simulink library "powerlib2"  (Simulink 6.0)
settings: Solver=ode45  SolverMode=SingleTasking  StartTime=0.0  StopTime=10.0  RelTol=1e-3
undefined symbols (not defined in the file or in its folder): com, ctrl1, Da, DiscIntNeverNeededParam, dtha, etat, FA, gcbh, Ha, Ka, Lm, Ls, powericonV2, q0, Rm, Rs, sel, st_a, st_b, st_c, sta, stb, stc, T1, T2, T3, T4
libraries: powerlib2 x55, simulink_extras x5, powerlib_extras x4, powerlib_modelsV2 x4, simulink x1
(part 3 of 6)

== system powerlib2/Machines ==
  note: ____ S y n c h r o n o u s M a c h i n e s ____________________
  note: ____ D C M a c h i n e s _______________________
  note: ____ A s y n c h r o n o u s M a c h i n e s ___________________
  note: ____ P r i m e M o v e r s a n d R e g u l a t o r s _____
  note: ____ M a c h i n e M e a s u r e m e n t s ___________
  Asynchronous Machine SI Units : Subsystem  Tag=PoWeRsYsTeMbLoCk  LoadFcn=powericonV2('psblfblk',bdroot,'gotofrom','Load');  mask(Asynchronous Machine){rotType=Wound, ctrl=Rotor, x1=[ 3*746, 220, 60 ], x2=[ 0.435  2.0e-3 ], x3=[ 0.816  2.0e-3 ], x4=69.31e-3, x5=[ 0.089  0  2 ], x6=[ 1,0   0,0,0   0,0,0 ], PSBOutputType=1110, iounits=1, LoadFlowParameters=0}
      mask prompts: rotType "Rotor type:"; ctrl "Reference frame:"; x1 "Nom. power,L-L volt. and freq. [ Pn(VA),Vn(Vrms),fn(Hz) ]:"; x2 "Stator [ Rs(ohm)  Lls(H) ]:"; x3 "Rotor [ Rr'(ohm)  Llr'(H) ]:"; x4 "Mutual inductance Lm (H):"; x5 "Inertia,friction factor and pairs of poles [ J(kg.m^2)  F(N.m.s)  p() ]:"; x6 "Initial conditions  (read the details in the description above)"; PSBOutputType "Output type [1=PSB  0=simulink output]"; LoadFlowParameters "Load flow Parameters"
      mask help:
      | Implements a three-phase asynchronous machine (wound rotor or squirrel cage) modeled in the dq rotor reference frame. Stator and rotor windings are connected in wye to an internal neutral point. Press help for inputs and outputs description.
      |
      | You can specify initial  values for stator and rotor currents. In the Initial conditions parameter you have the possibility to specify the stator current only :
      |
      | [ s() th(deg)  isa,isb,isc(p.u.)  pha,phb,phc(deg) ]:
      |
      | Or you can choose to enter the stator and the rotor initial currents:
      |
      | [ s() th(deg)  isa,isb,isc(p.u.)  pha,phb,phc(deg) ira,irb,irc(pu)  pha,phb,phc ]:
      mask init:
      | [circl1,circl2,a1,a2,b1,b2,c1,c2,d1,d2,e1,e2,f1,f2,i1,i2] = powericonV2('Asynchronous Machine',rotType);
      | powericonV2('psbcbasm',gcb);
      settings: CopyFcn=powericonV2('psblfblk',bdroot,'gotofrom','Copy');
      mask Help: web(psbhelp);
      mask StyleString: popup(Wound|Squirrel-cage),popup(Rotor|Stationary|Synchronous),edit,edit,edit,edit,edit,edit,edit,edit,edit
      mask Display: plot(-55,-65,55,65,circl1,circl2,a1,a2,b1,b2,c1,c2,d1,d2,e1,e2,f1,f2,i1,i2);
  Asynchronous Machine pu Units : Subsystem  Tag=PoWeRsYsTeMbLoCk  LoadFcn=powericonV2('psblfblk',bdroot,'gotofrom','Load');  mask(Asynchronous Machine){rotType=Wound, ctrl=Rotor, x1=[ 3*746, 220, 60 ], x2=[ 0.0201,0.0349 ], x3=[ 0.0377,0.0349 ], x4=1.2082, x5=[ 0.7065,0,2 ], x6=[ 1,0   0,0,0   0,0,0 ], PSBOutputType=1110, iounits=0, LoadFlowParameters=0}
      mask prompts: rotType "Rotor type:"; ctrl "Reference frame:"; x1 "Nom. power,L-L volt. and freq. [ Pn(VA),Vn(Vrms),fn(Hz) ]:"; x2 "Stator [ Rs,Lls ] (pu):"; x3 "Rotor [ Rr',Llr' ] (pu):"; x4 "Mutual inductance Lm (pu):"; x5 "Inertia constant,friction factor and pairs of poles [ H(s) F(pu) p() ]:"; x6 "Initial conditions  (read the details in the description above)"; PSBOutputType "Output type [1=PSB  0=simulink output]"; LoadFlowParameters "Load Flow Parameters"
      mask help:
      | Implements a three-phase asynchronous machine (wound rotor or squirrel cage) modelled in the dq rotor reference frame. Stator and rotor windings are connected in wye to an internal neutral point. Press help for inputs and outputs description.
      |
      | You can specify initial  values for stator and rotor currents. In the Initial conditions parameter you have the possibility to specify the stator current only :
      |
      | [ s() th(deg)  isa,isb,isc(p.u.)  pha,phb,phc(deg) ]:
      |
      | Or you can choose to enter the stator and the rotor initial currents:
      |
      | [ s() th(deg)  isa,isb,isc(p.u.)  pha,phb,phc(deg) ira,irb,irc(pu)  pha,phb,phc ]:
      mask init:
      | [circl1,circl2,a1,a2,b1,b2,c1,c2,d1,d2,e1,e2,f1,f2,i1,i2] = powericonV2('Asynchronous Machine',rotType);
      | powericonV2('psbcbasm',gcb);
      settings: CopyFcn=powericonV2('psblfblk',bdroot,'gotofrom','Copy');
      mask Help: web(psbhelp);
      mask StyleString: popup(Wound|Squirrel-cage),popup(Rotor|Stationary|Synchronous),edit,edit,edit,edit,edit,edit,edit,edit,edit
      mask Display: plot(-55,-65,55,65,circl1,circl2,a1,a2,b1,b2,c1,c2,d1,d2,e1,e2,f1,f2,i1,i2);
  DC Machine : Subsystem  mask(DC machine){RLa=[ 0.6  0.012], RLf=[ 240  120], Laf=1.8, J=1, Bm=0, Tf=0, w0=1, PSBOutputType=110}
      mask prompts: RLa "Armature resistance and inductance [Ra (ohms) La (H) ]"; RLf "Field resistance and inductance [Rf (ohms) Lf (H) ]"; Laf "Field-armature mutual inductance Laf (H) :"; J "Total inertia J (kg.m^2)"; Bm "Viscous friction coefficient Bm (N.m.s)"; Tf "Coulomb friction torque Tf (N.m)"; w0 "Initial speed (rad/s) :"; PSBOutputType "Output type"
      mask help:
      | This block implements a separately excited DC machine. Access is provided  to the field connections so that the machine can be used as a shunt-connected or a series-connected  DC machine.
      |
      | Input 1 and output 1 : positive and negative armature terminals
      | Input 2 and output 2 : positive and negative field terminals
      | Input 3    : Load torque
      | Output 3 : Simulink measurement output [ w Ia If Te ]
      mask init:
      | Ra=RLa(1); La=RLa(2);
      | Rf=RLf(1); Lf=RLf(2);
      mask Help: web(psbhelp)
      mask Display: plot(-80,-80,80,80,[0,9,18,24,29,30,29,24,18,9,0,-9,-18,-24,-29,-30,-29,-24,-18,-9,0],[30,29,24,18,9,0,-9,-18,-24,-29,-30,-29,-24,-18,-9,0,9,18,24,29,30],[-29,-35,-35,-29],[-8,-8,8,8],[29,35,35,29],[-8,-8,8,8],[-35,-55],[0,0],[35,55],[0,0],[-78,-50,-50,-49,-45,-39,-33,-26,-21,-18,-17,-19,-22,-22,-26,-27,-25,-22,-16,-9,-3,2,6,6,4,1,1,-3,-4,-2,2,7,14,20,26,29,30,28,24,24,21,20,21,25,31,37,44,49,50,50,50,78]*.7,[58,58,57.2,49.2,42.8,38.8,38,39.6,44.4,51.6,59.6,67.6,72.4,72.4,65.2,57.2,49.2,42.8,38.8,38,39.6,44.4,51.6,59.6,67.6,72.4,72.4,65.2,57.2,49.2,42.8,38.8,38,39.6,44.4,51.6,59.6,67.6,72.4,72.4,65.2,57.2,49.2,42.8,38.8,38,39.6,44.4,51.6,58,58,58]*.6+15 );
  Discrete DC_Machine : powerlib_extras/Additional Machines/Discrete DC_Machine  RLa="[0.5  0.01]"  RLf="[240  0]"  Laf=1.23  J=0.05  Bm=0.02  Tf=0  w0=0  PSBOutputType=110  Ts=50e-6
  Excitation System : Subsystem  InitFcn=powericonV2('psbcallbacks',gcb,'Excitationsystem',1);  mask(Excitation System){tr=20e-3, reg=[ 300, 0.001 ], exc=[ 1, 0 ], tgr=[ 0, 0 ], damp=[ 0.001, 0.1 ], sat=[ 0, 0 ], lim=[ -11.5, 11.5, 0 ], v0=[1.0  1.28]}
      mask prompts: tr "Low-pass filter time constant Tr(s):"; reg "Regulator gain and time constant [ Ka()  Ta(s) ]:"; exc "Exciter  [ Ke()  Te(s) ]:"; tgr "Transient gain reduction [ Tb(s)  Tc(s) ]:"; damp "Damping filter gain and time constant  [ Kf()  Tf(s)  ]:"; sat "Field saturation parameters [ A, B ]:"; lim "Regulator output limits and gain [ Efmin, Efmax (p.u.), Kp() ]:"; v0 "Initial values of terminal voltage  and field voltage [ Vt0 (pu) Vf0(pu) ] :"
      mask help:
      | Implements an IEEE type 1 synchronous machine voltage regulator combined to an exciter. This block uses the dq components of terminal voltage (Synchronous Machine block, measurement ouputs 9 and 10).
      |
      | 1st input: desired stator terminal voltage (p.u.);
      | 2nd input: vd component of the terminal voltage (p.u.);
      | 3rd input: vq component of the terminal voltage (p.u.);
      | 4th input: stabilization voltage from user-supplied
      |                  power system stabilizer (p.u.);
      |
      | output: field voltage vfd to be applied to the
      |              Synchronous Machine block's 2nd input (p.u.).
      mask init:
      | ka=reg(1);ta=reg(2);ke=exc(1);te=exc(2);tb=tgr(1);tc=tgr(2);kf=damp(1);tf=damp(2);efmin=lim(1);efmax=lim(2);a=sat(1);b=sat(2);kp=lim(3);
      mask Help: web(psbhelp);
  Generic Power System Stabilizer : Subsystem  InitFcn=powericonV2('psbcbtransfo',gcb,'PSS',1);  mask(Generic Power System Stabilizer){Tsensor=30e-3, K=20, Twashout=2, Tleadlag1=[50e-3 20e-3], Tleadlag2=[3 5.4], VSlimits=[-0.15 0.15], Vinit=0, Plot_On=off, MagdB_On=on, FreqRange=logspace(-2,2,500)}
      mask prompts: Tsensor "Sensor time constant:"; K "Gain:"; Twashout "Wash-out time constant:"; Tleadlag1 "Lead-lag #1 time constants: [ Tnum Tden ]"; Tleadlag2 "Leag-lag #2 time constants: [ Tnum Tden ]"; VSlimits "Output limits: [ VSmin VSmax ]"; Vinit "Initial input:"; Plot_On "Plot frequency response"; MagdB_On "Magnitude in dB"; FreqRange "Frequency range (Hz):"
      mask help:
      | This block implements a generic Power System Stabilizer (PSS).
      |
      | Input (In): Synchronous machine speed deviation with respect to nominal (dw in pu) or acceleration power (Pa=Pm-Pe in pu).
      | Output (VS): stabilization voltage (pu).
      |
      | Look under mask to see how the various transfer functions are connected.
      mask init:
      | T1n=Tleadlag1(1);
      | T1d=Tleadlag1(2);
      | T2n=Tleadlag2(1);
      | T2d=Tleadlag2(2);
      | %
      | if Plot_On==1,
      | % Compute global system (sysG):
      | numS=[1];
      | denS=[Tsensor 1];
      | sysS=tf(numS,denS);
      | numW=[Twashout 0];
      | denW=[Twashout 1];
      | sysW=tf(numW,denW);
      | numL1=[T1n 1];
      | denL1=[T1d 1];
      | sysL1=tf(numL1,denL1);
      | numL2=[T2n 1];
      | denL2=[T2d 1];
      | sysL2=tf(numL2,denL2);
      | sysG=sysS*K*sysW*sysL1*sysL2;
      | %
      | % Plot response:
      | w=2*pi*FreqRange;
      | [Mag,Pha]=bode(sysG,w);
      | subplot(2,1,1)
      | if  MagdB_On==1,
      | Y= 20*log10(squeeze(Mag)) ;
      | strLabel='dB';
      | else
      | Y=squeeze(Mag);
      | strLabel='pu/pu';
      | end
      | %
      | semilogx(FreqRange,Y)
      | ylabel(strLabel);grid;
      | title('PSS Frequency Response');
      | subplot(2,1,2);
      | semilogx(FreqRange,rem(squeeze(Pha),360))
      | ylabel('Degrees');grid;
      | xlabel('Frequency (Hz)');
      | end
      mask Help: web(psbhelp)
      mask CallbackString: |||||||parametres=get_param(gcb,'MaskValues');p8=parametres{8};if strcmp(p8,'on');param9='on';param10='on';else;param9='off';param10='off';end;visible={'on','on','on','on','on','on','on','on',param9,param10};set_param(gcb,'MaskVisibilities',visible)||
  HTG : Subsystem  InitFcn=powericonV2('psbcallbacks',gcb,'HTGsystem',1);  mask(Hydraulic Turbine and Governor){sm=[ 10/3  0.07 ], gate=[  0.01  0.97518  -0.1  0.1 ], reg=[  0.05  1.163  0.105  0  0.01  ], hyd=[  0  2.67  ], dref=0, po=0.7516}
      mask prompts: sm "Servo-motor [ Ka()  Ta(sec) ]:"; gate "Gate opening limits [ gmin,gmax(pu)    vgmin,vgmax(pu/s) ]:"; reg "Permanent droop and regulator  [ Rp() Kp() Ki() Kd() Td(s) ]:"; hyd "Hydraulic turbine [ beta()  Tw(sec) ]:"; dref "Droop reference (0=power error, 1=gate opening):"; po "Initial mechanical power (pu):"
      mask help:
      | Implements a hydraulic turbine combined to a PID governor system.
      |
      | 1st input: desired speed (p.u.);
      | 2nd input: desired electrical power (p.u.);
      | 3rd input: synchronous machine's actual speed (p.u., measurement output 13 of SM block);
      | 4th input: synchronous machine's actual electrical power (p.u., measurement output 14 of SM block);
      | 5th input: synchronous machine's actual speed deviation with respect to nominal (%, measurement output 15 of SM block);
      |
      | 1st output: mechanical power to be applied to the Synchronous Machine block's 1st input (p.u.);
      | 2nd output: gate opening (p.u.).
      mask init:
      | ka=sm(1);ta=sm(2);gmin=gate(1);gmax=gate(2);vgmin=gate(3);vgmax=gate(4);Rp=reg(1);kp=reg(2);ki=reg(3);kd=reg(4);td=reg(5);beta=hyd(1);tw=hyd(2);go=po*(gmax-gmin);
      mask Help: web(psbhelp);
  Machines Measurement Demux : Subsystem  mask(Machine measurements){machType=Synchronous, ssm1=on, ssm2=on, ssm3=on, ssm4=on, ssm5=on, ssm6=on, sm1=off, sm2=on, sm3=off, sm4=off, sm5=off, sm6=on, sm7=off, sm8=on, sm9=off, sm10=off, sm11=off, sm115=off, sm12=off, sm13=off, sm14=off, asm1=on, asm2=on, asm3=on, asm4=on, asm5=on, asm6=on, asm7=on, asm8=on, asm9=on, asm10=on, asm11=on, pmsm1=on, pmsm2=on, pmsm3=on, pmsm4=on, pmsm5=on, pmsm6=on, lastType=1}
      mask prompts: machType "Machine type:"; ssm1 "Line currents          [ isa  isb  isc ]"; ssm2 "Terminal voltages   [ va  vb  vc ]"; ssm3 "Internal voltages     [ ea  eb  ec ]"; ssm4 "Rotor angle            [ thetam ]   rad"; ssm5 "Rotor speed           [ wm ]"; ssm6 "Electrical power     [ Pe ]"; sm1 "Stator currents                  [ isa  isb  isc ]"; sm2 "Stator currents                  [ iq  id ]"; sm3 "Field current                      [ ifd ]"; sm4 "Damper winding currents   [ ikq1  ikq2  ikd ]"; sm5 "Mutual fluxes                     [ phim_q   phim_d ]"; sm6 "Stator voltages                  [ vs_q   vs_d ]"; sm7 "Rotor angle deviation        [ d_theta ]   rad"; sm8 "Rotor speed                       [ wm ]"; sm9 "Electrical power                 [ Pe ]"; sm10 "Rotor speed deviation       [ dw ]"; sm11 "Rotor mechanical angle     [ theta ]   deg"; sm115 "Electromagnetic torque     [ Te ]"; sm12 "Load angle                         [ Delta ]   deg"; sm13 "Output active power          [ Peo ]"; sm14 "Output reactive power       [ Qeo ]"; asm1 "Rotor currents    [ ira  irb  irc ]"; asm2 "Rotor currents    [ ir_q   ir_d  ]"; asm3 "Rotor fluxes       [ phir_q   phir_d ]"; asm4 "Rotor voltages   [ vr_q   vr_d ]"; asm5 "Stator currents   [ ia  ib  ic ]"; asm6 "Stator currents   [ is_q   is_d ]"; asm7 "Stator fluxes      [ phis_q  phis_d ]"; asm8 "Stator voltages   [ vs_q  vs_d ]"; asm9 "Rotor speed       [ wm ]"; asm10 "Electromagnetic torque  [Te ]  pu"; asm11 "Rotor angle        [ thetam ]  rad"; pmsm1 "Stator currents   [ ia, ib, ic ]  A"; pmsm2 "stator currents    [ is_q   is_d ]  A"; pmsm3 "Stator voltages   [ vs_q   vs_d ]   V"; pmsm4 "Rotor speed       [ wm ]   rad/s"; pmsm5 "Rotor angle        [ thetam ]  rad"; pmsm6 "Electromagnetic torque  [Te ]  N.m"
      mask help:
      | Split specified signals of various machine models measurement output vector into separate signals.
      | Set the "Machine units" parameter to the units used for the machine connected to the block input.
      mask init:
      | t = powericonV2('Machines Demux Model',gcb);
      mask StyleString: popup(Simplified synchronous|Synchronous|Asynchronous|Permanent magnet synchronous),checkbox,checkbox,checkbox,checkbox,checkbox,checkbox,checkbox,checkbox,checkbox,checkbox,checkbox,checkbox,checkbox,checkbox,checkbox,checkbox,checkbox,checkbox,checkbox,checkbox,checkbox,checkbox,checkbox,checkbox,checkbox,checkbox,checkbox,checkbox,checkbox,checkbox,checkbox,checkbox,checkbox,checkbox,checkbox,checkbox,checkbox,checkbox,edit
      mask CallbackString: powericonV2('psbcbmachdemux',gcb)|||||||||||||||||||||||||||||||||||||||
      mask Display: plot([0 0],[t t])
  Multi-Band Power System Stabilizer : Subsystem  InitFcn=powericonV2('psbcallbacks',gcb,'MBPSS',1);  mask(Multi-Band Power System Stabilizer ){OperationMode=Simplified settings, Kg=1.0, GL=[0.2 20], GI=[0.9 25], GH=[12.0 145], GLd=[66 66 9.4], TcLF=[1.667 2 0 0 0 0 2 2.4 0 0 0 0 1 1], GId=[66 66 47.6], TcIF=[1 1 0.25 0.3 0 0 1 1 0.3 0.36 0 0 0 0], GHd=[66 66 233], TcHF=[0.01 0.012 0 0 0 0  0.012 0.0144 0 0 0 0 1 1], LIM=[.075 .15 .15 .15], Plot_On=off, MagdB_On=off, FreqRange=logspace(-2,2,500)}
      mask prompts: OperationMode "Mode of operation:"; Kg "Global gain:"; GL "Low frequency band: [ FL(Hz), KL ]"; GI "Intermediate frequency band: [ FI(Hz), KI ]"; GH "High frequency band: [ FH(Hz), KH ]"; GLd "Low frequency gains: [ KL1, KL2, KL ]"; TcLF "Low frequency  time constants (s):"; GId "Intermediate frequency gains: [ KI1, KI2, KI ]"; TcIF "Intermediate frequency time constants (s):"; GHd "High frequency gains: [ KH1, KH2, KH ]"; TcHF "High frequency time constants (s):"; LIM "Signals Limits(VLmax,VImax,VHmax,VSmax)"; Plot_On "Plot frequency response"; MagdB_On "Magnitude in dB"; FreqRange "Frequency range (Hz):"
      mask help:
      | This block implements a Multi-band Power System Stabilizer (MB-PSS). Two operation modes are available: Detailed setting and simplified setting (IEEE Std 421.5).
      |
      | When "Detailed settings" is used, the low(L)-, intermediate(I)- and high(H)-frequency time constants must be given in the following order:
      | Tx1 to Tx12 followed by Kx11 and Kx17 (where x=L, I or H). Look under mask to see in which transfer functions these time constants are used.
      mask init:
      | Detailed=0;
      | if OperationMode==2,
      | Detailed=1;
      | Kg=1;
      | KL1=GLd(1);KL2=GLd(:,2);KL=GLd(3);
      | TL1=TcLF(1);TL2=TcLF(2);TL3=TcLF(3);TL4=TcLF(4);
      | TL5=TcLF(5);TL6=TcLF(6);TL7=TcLF(7);TL8=TcLF(8);
      | TL9=TcLF(9);TL10=TcLF(10);TL11=TcLF(11);TL12=TcLF(12);
      | KL11=TcLF(13);KL17=TcLF(14);
      | KI1=GId(1);KI2=GId(:,2);KI=GId(3);
      | TI1=TcIF(1);TI2=TcIF(2);TI3=TcIF(3);TI4=TcIF(4);
      | TI5=TcIF(5);TI6=TcIF(6);TI7=TcIF(7);TI8=TcIF(8);
      | TI9=TcIF(9);TI10=TcIF(10);TI11=TcIF(11);TI12=TcIF(12);
      | KI11=TcIF(13);KI17=TcIF(14);
      | KH1=GHd(1);KH2=GHd(:,2);KH=GHd(3);
      | TH1=TcHF(1);TH2=TcHF(2);TH3=TcHF(3);TH4=TcHF(4);
      | TH5=TcHF(5);TH6=TcHF(6);TH7=TcHF(7);TH8=TcHF(8);
      | TH9=TcHF(9);TH10=TcHF(10);TH11=TcHF(11);TH12=TcHF(12);
      | KH11=TcHF(13);KH17=TcHF(14);
      | else
      | %
      | R=1.2;K=(R*R+R)/(R*R-2*R+1);KL1=K;KL2=K;KI1=K;KI2=K;KH1=K;KH2=K;
      | TL2=1/(2*pi*GL(1)*sqrt(R));KL=GL(2);TL1=TL2/R;TL7=TL2;TL8=TL7*R;
      | %
      | TI2=1/(2*pi*GI(1)*sqrt(R));KI=GI(2);TI1=TI2/R;TI7=TI2;TI8=TI7*R;
      | TH2=1/(2*pi*GH(1)*sqrt(R));KH=GH(2);TH1=TH2/R;TH7=TH2;TH8=TH7*R;
      | %
      | TL3=0;TL4=0;TL5=0;TL6=0;TL9=0;TL10=0;TL11=0;TL12=0;
      | TI3=0;TI4=0;TI5=0;TI6=0;TI9=0;TI10=0;TI11=0;TI12=0;
      | TH3=0;TH4=0;TH5=0;TH6=0;TH9=0;TH10=0;TH11=0;TH12=0;
      | KL11=1;KL17=1;KI11=1;KI17=1;KH11=1;KH17=1;
      | end
      | LIM_VL=LIM(1);LIM_VI=LIM(2);LIM_VH=LIM(3);LIM_VS=LIM(4);
      | %
      | % LF Transfer function
      | numLF1=[TL1 KL11];
      | denLF1=[TL2 1];
      | sysLF1=tf(numLF1,denLF1);
      | numLF2=[TL3 1];
      | denLF2=[TL4 1];
      | sysLF2=tf(numLF2,denLF2);
      | numLF3=[TL5 1];
      | denLF3=[TL6 1];
      | sysLF3=tf(numLF3,denLF3);
      | numLF4=[TL7 KL17];
      | denLF4=[TL8 1];
      | sysLF4=tf(numLF4,denLF4);
      | numLF5=[TL9 1];
      | denLF5=[TL10 1];
      | sysLF5=tf(numLF5,denLF5);
      | numLF6=[TL11 1];
      | denLF6=[TL12 1];
      | sysLF6=tf(numLF6,denLF6);
      | %
      | sysLF=Kg*KL*((KL1*sysLF1*sysLF2*sysLF3) - (KL2*sysLF4*sysLF5*sysLF6));
      | %
      | %
      | % IF transfer function
      | numIF1=[TI1 KI11];
      | denIF1=[TI2 1];
      | sysIF1=tf(numIF1,denIF1);
      | numIF2=[TI3 1];
      | denIF2=[TI4 1];
      | sysIF2=tf(numIF2,denIF2);
      | numIF3=[TI5 1];
      | denIF3=[TI6 1];
      | sysIF3=tf(numIF3,denIF3);
      | numIF4=[TI7 KI17];
      | denIF4=[TI8 1];
      | sysIF4=tf(numIF4,denIF4);
      | numIF5=[TI9 1];
      | denIF5=[TI10 1];
      | sysIF5=tf(numIF5,denIF5);
      | numIF6=[TI11 1];
      | denIF6=[TI12 1];
      | sysIF6=tf(numIF6,denIF6);
      | %
      | sysIF=Kg*KI*((KI1*sysIF1*sysIF2*sysIF3) - (KI2*sysIF4*sysIF5*sysIF6));
      | %
      | %
      | % HF transfer function
      | numHF1=[TH1 KH11];
      | denHF1=[TH2 1];
      | sysHF1=tf(numHF1,denHF1);
      | numHF2=[TH3 1];
      | denHF2=[TH4 1];
      | sysHF2=tf(numHF2,denHF2);
      | numHF3=[TH5 1];
      | denHF3=[TH6 1];
      | sysHF3=tf(numHF3,denHF3);
      | numHF4=[TH7 KH17];
      | denHF4=[TH8 1];
      | sysHF4=tf(numHF4,denHF4);
      | numHF5=[TH9 1];
      | denHF5=[TH10 1];
      | sysHF5=tf(numHF5,denHF5);
      | numHF6=[TH11 1];
      | denHF6=[TH12 1];
      | sysHF6=tf(numHF6,denHF6);
      | %
      | sysHF=Kg*KH*((KH1*sysHF1*sysHF2*sysHF3) - (KH2*sysHF4*sysHF5*sysHF6));
      | %
      | %
      | % Input filter LIF
      | numLIFin=[1.759e-3 1];
      | denLIFin=[1.2739e-4 1.7823e-2 1];
      | sysLIFin=tf(numLIFin,denLIFin);
      | % Input filter HF
      | numHFin=[80 0 0];
      | denHFin=[1 82 161 80];
      | sysHFin=tf(numHFin,denHFin);
      | %
      | % Global transfer function:
      | sysL=sysLIFin*sysLF;
      | sysI=sysLIFin*sysIF;
      | sysH=sysHFin*sysHF;
      | sysG=sysL+sysI + sysH;
      | %
      | % Plot frequency response:
      | if Plot_On==1,
      |     w=2*pi*FreqRange;
      |     [MagL,PhaseL]=bode(sysL,w);
      |     [MagI,PhaseI]=bode(sysI,w);
      |     [MagH,PhaseH]=bode(sysH,w);
      |     [MagG,PhaseG]=bode(sysG,w);
      |     subplot(2,1,1)
      |      if  MagdB_On==1,
      |         YL= 20*log10(squeeze(MagL)) ;
      |         YI= 20*log10(squeeze(MagI)) ;
      |         YH= 20*log10(squeeze(MagH)) ;
      |         YG= 20*log10(squeeze(MagG)) ;
      |          strLabel='dB';
      | else
      | YL=squeeze(MagL);
      | YI=squeeze(MagI);
      | YH=squeeze(MagH);
      | YG=squeeze(MagG);
      | strLabel='pu/pu';
      | end
      | semilogx(FreqRange,YL,'m',FreqRange,YI,'g',FreqRange,YH,'b',FreqRange,YG,'r')
      | ylabel(strLabel);grid;
      | legend('LF band','IF band','HF band','Global',2);
      | title('PSS Frequency Response');
      |  subplot(2,1,2);
      | semilogx(FreqRange,rem(squeeze(PhaseL),360),'m',FreqRange,rem(squeeze(PhaseI),360),'g',FreqRange,rem(squeeze(PhaseH),360),'b',FreqRange,rem(squeeze(PhaseG),360),'r');
      | ylabel('Degrees');grid;
      | xlabel('Frequency (Hz)');
      | end
      settings: CopyFcn=powericonV2('psbcbtransfo',gcb,'MBPSS',2);
      mask Help: web(psbhelp)
      mask StyleString: popup(Simplified settings|Detailed settings),edit,edit,edit,edit,edit,edit,edit,edit,edit,edit,edit,checkbox,checkbox,edit
      mask CallbackString: powericonV2('psbcbtransfo',gcb,'MBPSSmodel',1);||||||||||||parametres=get_param(gcb,'MaskValues');p1=parametres{1};p13=parametres{13};if strcmp(p1,'Detailed settings');param2='off';param3='off';param4='off';param5='off';param6='on';param7='on';param8='on';param9='on';param10='on';param11='on';else;param2='on';param3='on';param4='on';param5='on';param6='off';param7='off';param8='off';param9='off';param10='off';param11='off';end;if strcmp(p13,'on');param14='on';param15='on';else;param14='off';param15='off';end;visible={'on',param2,param3,param4,param5,param6,param7,param8,param9,param10,param11,'on','on',param14,param15};set_param(gcb,'MaskVisibilities',visible)||
  Permanent Magnet Synchronous Machine : Subsystem  Tag=PoWeRsYsTeMbLoCk  LoadFcn=powericonV2('psblfblk',bdroot,'gotofrom','Load');  mask(PM Synchronous Machine){x1=2.8750, x2=[8.5e-3, 8.5e-3], x3=0.175, x4=[ 0.8e-3, 0,  4 ], PSBOutputType=0}
      mask prompts: x1 "Resistance R(ohm):"; x2 "Inductances [ Ld(H) Lq(H) ]:"; x3 "Flux induced by magnets (Wb):"; x4 "Inertia, friction factor and pairs of poles [ J(kg.m^2)  F(N.m.s)  p() ]:"; PSBOutputType "Output type [1=PSB  0=simulink output]"
      mask help:
      | Implements a 3-phase permanent magnet synchronous machine with sinusoidal flux distribution. The machine is modelled in the dq rotor reference frame. Stator windings are connected in wye to an internal neutral point.
      |
      | First 3 inputs: Machine terminals =  phases a, b and c
      | 4th input:  Simulink signal = mechanical torque (N.m)
      |                    (>0 for motor mode,<0 for generator mode)
      |
      | output: Simulink measurement output = vector (10x1) containing
      |              (all currents flowing into machine):
      |   1-3 : Stator line currents ia, ib, ic (A)
      |   4-5 : Stator currents iq, id (A)
      |   6-7 : Stator voltages vq, vd (V)
      |   8     : Rotor speed wm (rad/s)
      |   9     : Rotor angle thetam (rad)
      |   10   : Electromagnetic torque Te (N.m)
      mask init:
      | [circl1,circl2,a1,a2,b1,b2,c1,c2,d1,d2,n1,n2,s1,s2] = powericonV2('PM Synchronous Machine');
      settings: CopyFcn=powericonV2('psblfblk',bdroot,'gotofrom','Copy');
      mask Help: web(psbhelp);
      mask Display: plot(-60,-60,60,60,circl1,circl2,a1,a2,b1,b2,c1,c2,d1,d2,n1,n2,s1,s2);
  STG : Subsystem  mask(Steam Turbine and Governor){gentype=Tandem-compound (multi-mass), reg1=[ 1  0.05    0 ], reg2=[ 0.001  0.15 ], reg3=[ -0.1  0.1  0  4.496 ], turb1=[ 0  10   3.3   0.5   ], turb2=[   0   0.36    0.36   0.28   ], HA=[ 0.046  1.430  1.465   0.192 ], KA=[ 90.44  53.88  64.59   62.94  ], DA=[ 0.0115  0.3575  0.3663   0.0137  ], ini1=250.35/555, ini2=[ 250.35/555   -51.2424   ]}
      mask prompts: gentype "Generator type"; reg1 "Regulator gain, perm. droop, dead zone [ Kp  Rp(p.u.)  Dz(p.u.) ]:"; reg2 "Speed relay and servo-motor time constants [ Tsr  Tsm ] (s):"; reg3 "Gate opening limits [ vgmin,vgmax (p.u./s)  gmin,gmax (p.u.)]:"; turb1 "Steam turbine time constants [ T2  T3  T4  T5 ] (s):"; turb2 "Turbine torque fractions [ F2  F3  F4  F5 ]:"; HA "Coeff. of inertia [ H2  H3  H4  H5 ] (s):"; KA "Stiffness coeff. [ K12  K23  K34  K45 ] (pu/rad):"; DA "Damping factors [ D2  D3  D4  D5 ] (p.u. T/p.u. dw):"; ini1 "Initial power Pm0 (p.u.):"; ini2 "Initial power and generator rotor angle [ Pm0 (p.u.)  th0(deg) ]:"
      mask help:
      | Implements a complete tandem-compound steam prime mover system, including speed regulator, steam turbine and a shaft with up to 4 masses. The genererator's mass is labelled mass #1 and is not included here. The shaft mass closest to the generator is #2, the farthest is #5. If a mass is not to be included, set it's inertia H to zero. The damping factor and rigidity coefficients corresponding to omitted masses are not considered and can be left as is. When masses are omitted, the remaining system is "compressed" towards the generator i.e. if only 2 masses are used, it will be masses #2 and #3. The input data for the masses considered is shifted accordingly.
      |
      | Press Help for inputs and outputs description.
      mask init:
      | if gentype==1, HA=[];DA=[];KA=[]; ini2=[]; end
      | 
      | [q0,FA,Ha,Ka,Da,dtha,t,errorFlag,ctrl1,sel,massNumber] = powericonV2(...
      | 'STG Model',gentype,reg1,reg2,reg3,turb1,turb2,HA,KA,DA,ini1,ini2);
      | 
      | switch errorFlag
      | case 1, error('Torque fractions total (gen.A)  is not 1 p.u.');
      | case 3
      |     mess=['You requested the multi-mass shaft but set all mass inertia',...
      |         ' constants to zero. Please use the single-mass option.'];
      |     error(mess);
      | case 4
      |    mess=['Inconsistent mass inertias and power fractions. Mass #',...
      |             num2str(massNumber),' has inertia set to zero but the ',...
      |             'corresponding torque fraction is not zero.'];
      |     error(mess);
      | case 5
      |         error('Parameters error');
      | end
      mask Help: web(psbhelp);
      mask StyleString: popup(Tandem-compound (single mass)|Tandem-compound (multi-mass)),edit,edit,edit,edit,edit,edit,edit,edit,edit,edit
      mask CallbackString: powericonV2('psbcbstg',gcb)||||||||||
      mask Display: plot([0 0],[t t])
  Simplified Synchronous  Machine  pu Units : Subsystem  Tag=PoWeRsYsTeMbLoCk  LoadFcn=powericonV2('psblfblk',bdroot,'gotogotofrom','Load');  mask(Simplified Synchronous Machine){conType=3-wire Y, x1=[ 1000e6,315e3,60 ], x2=[ inf,0,2 ], x3=[ 0.02,1 ], x4=[ 0   0   0,0,0   0,0,0 ], PSBOutputType=1111, iounits=0, LoadFlowParameters=[1,0,0,0,0]}
      mask prompts: conType "Connection type:"; x1 "Nom. power, L-L volt., and freq. [ Pn(VA) Vn(Vrms) fn(Hz) ]:"; x2 "Inertia, damping factor and pairs of poles[ H(sec)  Kd() p() ]:"; x3 "Internal impedance [ R(pu)  X(pu) ]:"; x4 "Init. cond. [ dw(%)  th(deg)  ia,ib,ic(pu)  pha,phb,phc(deg) ]:"; PSBOutputType "Output type [1=PSB  0=simulink output]"; LoadFlowParameters "Load Flow Parameters"
      mask help:
      | Implements a 3-phase simplified synchronous machine. Machine is modelled as an internal voltage behind a R-L impedance. Stator windings are connected in wye to an internal neutral point.
      |
      | 1st input: Simulink signal:  mechanical power supplied to the machine
      |                (p.u.,>0 for generator mode, <0 for motor mode)
      | 2nd input: Simulink signal: internal voltage (p.u.)
      |
      | First 3 outputs: Machine terminals = phases a, b and c
      | 4th output: Simulink measurement output = vector (12x1) containing :
      |    1-3 : Line currents flowing out of machine ia, ib, ic (p.u.)
      |    4-6 : Terminal voltages va, vb, vc (p.u.)
      |    7-9 : Internal voltages ea, eb, ec (p.u.)
      |    10   : Rotor angle theta (rad)
      |    11   : Rotor speed wm (p.u.)
      |    12   : Electrical power Pe (p.u.)
      mask init:
      | powericonV2('psbcbssm',gcb);
      settings: CopyFcn=powericonV2('psblfblk',bdroot,'gotogotofrom','Copy');
      mask Help: web(psbhelp);
      mask StyleString: popup(3-wire Y|4-wire Y),edit,edit,edit,edit,edit,edit,edit
      mask CallbackString: powericonV2('psbcbssm',gcb);|||||||
      mask Display: plot(-60,-60,60,60,[0,9,18,24,29,30,29,24,18,9,0,-9,-18,-24,-29,-30,-29,-24,-18,-9,0],[30,29,24,18,9,0,-9,-18,-24,-29,-30,-29,-24,-18,-9,0,9,18,24,29,30],[26,38],[15,15],[31,38],[0,0],[26,38],[-15,-15])
  Simplified Synchronous  Machine SI Units : Subsystem  Tag=PoWeRsYsTeMbLoCk  LoadFcn=powericonV2('psblfblk',bdroot,'gotogotofrom','Load');  mask(Simplified Synchronous Machine){conType=3-wire Y, x1=[ 1000e6,315e3,60 ], x2=[ inf,0,2 ], x3=[ 1.9845,263.15e-3 ], x4=[ 0   0   0,0,0   0,0,0 ], PSBOutputType=1111, iounits=1, LoadFlowParameters=[1,0,0,0,0]}
      mask prompts: conType "Connection type:"; x1 "Nom. power, L-L volt., and freq. [ Pn(VA) Vn(Vrms) fn(Hz) ]:"; x2 "Inertia, damping factor and pairs of poles[ J(kg.m^2)  Kd() p() ]:"; x3 "Internal impedance [ R(ohm)  L(H) ]:"; x4 "Init. cond. [ dw(%)  th(deg)  ia,ib,ic(A)  pha,phb,phc(deg) ]:"; PSBOutputType "Output type [1=PSB  0=simulink output]"; LoadFlowParameters "Load Flow Parameters"
      mask help:
      | Implements a 3-phase simplified synchronous machine. Machine is modelled as an internal voltage behind a R-L impedance. Stator windings are connected in wye to an internal neutral point.
      |
      | 1st input: Simulink signal:  mechanical power supplied to the machine
      |                  (W,>0 for generator mode, <0 for motor mode)
      | 2nd input: Simulink signal: RMS value of phase-to-phase internal voltage (V)
      |
      | First 3 outputs: Machine terminals = phases a, b and c
      | 4th output: Simulink measurement output = vector (12x1) containing :
      |    1-3 : Line currents flowing out of machine ia, ib, ic (A)
      |    4-6 : Terminal voltages va, vb, vc (V)
      |    7-9 : Internal voltages ea, eb, ec (V)
      |    10   : Rotor angle theta (rad)
      |    11   : Rotor speed wm (rad/s)
      |    12   : Electrical power Pe (W)
      mask init:
      | powericonV2('psbcbssm',gcb);
      settings: CopyFcn=powericonV2('psblfblk',bdroot,'gotogotofrom','Copy');
      mask Help: web(psbhelp);
      mask StyleString: popup(3-wire Y|4-wire Y),edit,edit,edit,edit,edit,edit,edit
      mask CallbackString: powericonV2('psbcbssm',gcb);|||||||
      mask Display: plot(-60,-60,60,60,[0,9,18,24,29,30,29,24,18,9,0,-9,-18,-24,-29,-30,-29,-24,-18,-9,0],[30,29,24,18,9,0,-9,-18,-24,-29,-30,-29,-24,-18,-9,0,9,18,24,29,30],[26,38],[15,15],[31,38],[0,0],[26,38],[-15,-15])
  Synchronous Machine SI Fundamental : Subsystem  Tag=PoWeRsYsTeMbLoCk  LoadFcn=powericonV2('psblfblk',bdroot,'gotogotofrom','Load');  mask(Synchronous Machine){rotorType=Salient-pole, x1=[ 187E6  13800   60   1087 ], x2=[ 2.9069E-03  3.0892E-04  3.2164E-03  9.7153E-04 ], x3=[ 5.9013E-04  3.0712E-04 ], x4b=[ 0.0664, 1.387e-3, 0.0292, 6.896e-4, 7.907e-3, 2.477e-3], x4=[ 1.1900E-02  4.9076E-04  2.0081E-02  1.0365E-03 ], x5=[ 3.895e6 0  20 ], x6=[ 0  0  0  0  0  0  0  0  70.3192 ], x7=off, x8=[695.64,774.7,917.5,1001.6,1082.2,1175.9,1293.6,1430.2,1583.7;9660,10623,12243,13063,13757,14437,15180,15890,16567], x9=off, PSBOutputType=1110, iounits=1, LoadFlowParameters=[1,0,0,0,0]}
      mask prompts: rotorType "Rotor type:"; x1 "Nom. power, volt., freq. and field cur. [ Pn(VA) Vn(Vrms) fn(Hz) ifn(A) ]:"; x2 "Stator [ Rs(ohm)  Ll,Lmd,Lmq(H) ]:"; x3 "Field [ Rf'(ohm)  Llfd'(H) ]:"; x4b "Dampers [ Rkd',Llkd'  Rkq1',Llkq1'  Rkq2',Llkq2'  ] (R=ohm,L=H):"; x4 "Dampers [ Rkd',Llkd'  Rkq1',Llkq1'  ] (R=ohm,L=H):"; x5 "Inertia, friction factor and pole pairs [ J(kg.m^2)  F(N.m.s)  p() ]:"; x6 "Init. cond. [ dw(%)  th(deg)  ia,ib,ic(A)  pha,phb,phc(deg)  Vf(V) ]:"; x7 "Simulate saturation"; x8 "Saturation parameters [ ifd1,ifd2,... (A) ; vt1,vt2,... (VLL rms) ]:"; x9 "Display Vfd which produces nominal Vt"; PSBOutputType "Output type [1=PSB  0=simulink output]"; LoadFlowParameters "Load Flow Parameters"
      mask help: Implements a 3-phase synchronous machine modelled in the dq rotor reference frame. Stator windings are connected in wye to an internal neutral point. Press help for inputs and outputs description.
      mask init:
      | circl1=[0,9,18,24,29,30,29,24,18,9,0,-9,-18,-24,-29,-30,-29,-24,-18,-9,0]*1.2;
      | circl2=[30,29,24,18,9,0,-9,-18,-24,-29,-30,-29,-24,-18,-9,0,9,18,24,29,30]*1.2;
      | i1 = [0,-9,-18,-24,-16,-16,-24,-18,-9,0,9,18,24,16,16,24,18,9,0];
      | i2 = [-30,-29,-24,-18,-18,18,18,24,29,30,29,24,18,18,-18,-18,-24,-29,-30]+15;
      | circl2=circl2+15;
      | a1 = [23,48];
      | a2 = [27,27]+15;
      | b1 = [36,48];
      | b2 = [15,15];
      | c1 = [23,48];
      | c2 = [-27,-27]+15;
      | d1 = [-36,-45,-45,60];
      | d2 = [0,0,-50,-50];
      settings: CopyFcn=powericonV2('psblfblk',bdroot,'gotogotofrom','Copy');
      mask Help: web(psbhelp);
      mask StyleString: popup(Salient-pole|Round),edit,edit,edit,edit,edit,edit,edit,checkbox,edit,checkbox,edit,edit,edit
      mask CallbackString: powericonV2('psbcbsyncmach',gcb)||||||||powericon('psbcbsyncmach',gcb)||powericonV2('psbcbsyncmach',gcb,1)|||
      mask Display: plot(-60,-60,60,60,circl1,circl2,a1,a2,b1,b2,c1,c2,i1,i2);
  Synchronous Machine pu Fundamental : Subsystem  Tag=PoWeRsYsTeMbLoCk  LoadFcn=powericonV2('psblfblk',bdroot,'gotogotofrom','Load');  mask(Synchronous Machine){rotorType=Salient-pole, x1=[ 187E6  13800   60 ], x2=[ 2.85E-03  0.114  1.19  0.36 ], x3=[ 5.79E-04  0.114], x4b=[0.0652, 0.5134, 0.0287, 0.2553, 7.765e-3, 0.9167 ], x4=[ 1.17E-02  0.182  1.97E-02  0384 ], x5=[ 3.7 0  20 ], x6=[ 0  0  0  0  0  0  0  0  1 ], x7=off, x8=[0.6404,0.7127,0.8441,0.9214,0.9956,1.082,1.19,1.316,1.457;0.7,0.7698,0.8872,0.9466,0.9969,1.046,1.1,1.151,1.201], PSBOutputType=1110, iounits=0, LoadFlowParameters=[1,0,0,0,0]}
      mask prompts: rotorType "Rotor type:"; x1 "Nom. power, L-L volt. and freq. [ Pn(VA)  Vn(Vrms)  fn(Hz) ]:"; x2 "Stator [ Rs  Ll  Lmd  Lmq ] (pu):"; x3 "Field [ Rf  Llfd ] (pu):"; x4b "Dampers [ Rkd,Llkd  Rkq1,Llkq1 Rkq2,Llkq2 ] (pu):"; x4 "Dampers [ Rkd,Llkd  Rkq1,Llkq1 ] (pu):"; x5 "Coeff. of inertia, friction factor and pole pairs [ H(s)  F(pu)  p() ]:"; x6 "Init. cond. [ dw(%)  th(deg)  ia,ib,ic(pu)  pha,phb,phc(deg)  Vf(pu) ]:"; x7 "Simulate saturation"; x8 "Saturation parameters [ ifd1,ifd2,... (p.u.) ; vt1,vt2,... (p.u.) ]:"; PSBOutputType "Output type [1=PSB  0=simulink output]"; LoadFlowParameters "Load Flow Parameters"
      mask help: Implements a 3-phase synchronous machine modelled in the dq rotor reference frame. Stator windings are connected in wye to an internal neutral point. Press help for inputs and outputs description.
      mask init:
      | circl1=[0,9,18,24,29,30,29,24,18,9,0,-9,-18,-24,-29,-30,-29,-24,-18,-9,0]*1.2;
      | circl2=[30,29,24,18,9,0,-9,-18,-24,-29,-30,-29,-24,-18,-9,0,9,18,24,29,30]*1.2;
      | i1 = [0,-9,-18,-24,-16,-16,-24,-18,-9,0,9,18,24,16,16,24,18,9,0];
      | i2 = [-30,-29,-24,-18,-18,18,18,24,29,30,29,24,18,18,-18,-18,-24,-29,-30]+15;
      | circl2=circl2+15;
      | a1 = [23,48];
      | a2 = [27,27]+15;
      | b1 = [36,48];
      | b2 = [15,15];
      | c1 = [23,48];
      | c2 = [-27,-27]+15;
      | d1 = [-36,-45,-45,60];
      | d2 = [0,0,-50,-50];
      | x9=0;
      settings: CopyFcn=powericonV2('psblfblk',bdroot,'gotogotofrom','Copy');
      mask Help: web(psbhelp);
      mask StyleString: popup(Salient-pole|Round),edit,edit,edit,edit,edit,edit,edit,checkbox,edit,edit,edit,edit
      mask CallbackString: powericonV2('psbcbsyncmach',gcb)||||||||powericon('psbcbsyncmach',gcb)||||
      mask Display: plot(-60,-60,60,60,circl1,circl2,a1,a2,b1,b2,c1,c2,i1,i2);
  Synchronous Machine pu Standard : Subsystem  Tag=PoWeRsYsTeMbLoCk  LoadFcn=powericonV2('psblfblk',bdroot,'gotogotofrom','Load');  mask(Synchronous Machine){rotorType=Salient-pole, x1=[ 187E6  13800   60 ], x2b=[ 1.81, 0.3, 0.23, 1.76, 0.65, 0.25, 0.15 ], x2=[ 1.305, 0.296, 0.252, 0.474, 0.243, 0.18 ], dAxisT=Open-circuit, qAxisT=Short-circuit, x3a=[ 4.4849  0.0681  0.1  ], x3b=[ 8.0, 0.03, 1.0, 0.07 ], x3c=[  4.49  0.0681  0.0513  ], x3d=[ 8.0, 0.03, 0.3371, 0.0295 ], x3=[ 1.01, 0.053, 0.1 ], x3e=[ 1.3201, 0.023, 1.0, 0.07 ], x3f=[  1.01  0.053  0.051266  ], x3g=[ 1.3201, 0.0231, 0.3371, 0.0295 ], x4=0.003, x5=[ 3.7 0  20 ], x6=[ 0  0  0  0  0  0  0  0  1 ], x7=off, x8=[0.6404,0.7127,0.8441,0.9214,0.9956,1.082,1.19,1.316,1.457;0.7,0.7698,0.8872,0.9466,0.9969,1.046,1.1,1.151,1.201], PSBOutputType=1110, iounits=0.5, LoadFlowParameters=[1,0,0,0,0]}
      mask prompts: rotorType "Rotor type:"; x1 "Nom. power, L-L volt. and freq. [ Pn(VA)  Vn(Vrms)  fn(Hz) ]:"; x2b "Reactances [ Xd Xd' Xd'' Xq Xq'  Xq'' Xl ] (pu):"; x2 "Reactances [ Xd Xd' Xd'' Xq Xq'' Xl ] (pu):"; dAxisT "d axis time constants:"; qAxisT "q axis time constant(s):"; x3a "Time constants [ Tdo'  Tdo''  Tqo'' ] (s):"; x3b "Time constants [ Tdo'  Tdo''  Tqo'  Tqo'' ] (s):"; x3c "Time constants [ Tdo'  Tdo''  Tq'' ] (s):"; x3d "Time constants [ Tdo'  Tdo''  Tq'  Tq'' ] (s):"; x3 "Time constants [ Td'  Td''  Tqo'' ] (s):"; x3e "Time constants [ Td'  Td''  Tqo'  Tqo'' ] (s):"; x3f "Time constants [ Td'  Td''  Tq'' ] (s):"; x3g "Time constants [ Td'  Td''  Tq'  Tq'' ] (s):"; x4 "Stator resistance Rs (p.u.):"; x5 "Coeff. of inertia, friction factor and pole pairs [ H(s)  F(pu)  p() ]:"; x6 "Init. cond. [ dw(%)  th(deg)  ia,ib,ic(pu)  pha,phb,phc(deg)  Vf(pu) ]:"; x7 "Simulate saturation"; x8 "Saturation parameters [ ifd1,ifd2,... (p.u.) ; vt1,vt2,... (p.u.) ]:"; PSBOutputType "Output type [1=PSB  0=simulink output]"; LoadFlowParameters "Load Flow Parameters"
      mask help: Implements a 3-phase synchronous machine modelled in the dq rotor reference frame. Stator windings are connected in wye to an internal neutral point. Press help for inputs and outputs description.
      mask init: same as powerlib2/Machines/Synchronous Machine pu Fundamental
      settings: CopyFcn=powericonV2('psblfblk',bdroot,'gotogotofrom','Copy');
      mask Help: web(psbhelp);
      mask StyleString: popup(Salient-pole|Round),edit,edit,edit,popup(Open-circuit|Short-circuit),popup(Open-circuit|Short-circuit),edit,edit,edit,edit,edit,edit,edit,edit,edit,edit,edit,checkbox,edit,edit,edit,edit
      mask CallbackString: powericonV2('psbcbsyncmach',gcb)||||powericonV2('psbcbsyncmach',gcb)|powericonV2('psbcbsyncmach',gcb)|||powericonV2('psbcbsyncmach',gcb)|||||||||powericonV2('psbcbsyncmach',gcb)||||
      mask Display: plot(-60,-60,60,60,circl1,circl2,a1,a2,b1,b2,c1,c2,i1,i2);

== system powerlib2/Measurements ==
  note: ____ E l e c t r i c a l ______________________________________
  note: _____ E x t r a M e a s u r e m e n t s ________________________
  Current Measurement : Subsystem  Tag=PoWeRsYsTeMmEaSuReMeNt  LoadFcn=powericonV2('psblcfmeas',gcb)  InitFcn=powericonV2('checksum',bdroot)  mask(Current Measurement){PhasorSimulation=off, OutputType=Magnitude, PSBOutputType=01, PSBequivalent=0}
      mask prompts: PhasorSimulation "Phasor simulation"; OutputType "Output signal :"; PSBOutputType "Output type [1=PSB  0=simulink output]"; PSBequivalent "Equivalentcircuit"
      mask help: Ideal current measurement.
      mask init:
      | switch OutputType
      | case 1
      |     OutputSelection = 1;
      |     NormalMode = 2;
      |     PhasorMode = 1;
      | case 2
      |     OutputSelection =[2,3];
      |     NormalMode = 3;
      |     PhasorMode = [1,2];
      | case 3
      |     OutputSelection =[4,5];
      |     NormalMode = 3;
      |     PhasorMode = [1,2];
      | case 4
      |     OutputSelection =[4];
      |     NormalMode = 2;
      |     PhasorMode = 1;
      | end
      | %
      | if PhasorSimulation
      |     SelectionMode = PhasorMode;
      | else
      |     SelectionMode = NormalMode;
      | end
      settings: CopyFcn=powericonV2('psblcfmeas',gcb,1)  ModelCloseFcn=powericonV2('loadsavedata',gcs,'close')
      mask Help: web(psbhelp);
      mask StyleString: checkbox,popup(Complex|Real-Imag|Magnitude-Angle|Magnitude),edit,edit
  "Extra Library " : Subsystem
      settings: OpenFcn=sys=sprintf('%s\n%s','powerlib_extras/Discrete','Measurements');powerlib_extras([],[],[],'load');open_system(sys)
      mask Display: disp(['Discrete\n Measurement\n blocks'])
  Extra Library 1 : Subsystem
      settings: OpenFcn=sys=sprintf('%s','powerlib_extras/Measurements');powerlib_extras([],[],[],'load');open_system(sys)
      mask Display: disp(['Measurement\n blocks'])
  Impedance Measurement : Subsystem  Tag=PoWeRsYsTeMbLoCk  mask(Impedance Measurement){kz=1}
      mask prompts: kz "Multiplication factor"
      mask help: Measure the impedance between two nodes of a circuit as a function of the frequency. Use the Powergui block to display the impedance calculation.
      settings: ModelCloseFcn=powericonV2('loadsavedata',gcs,'close')
      mask Help: web(psbhelp);
      mask Display: disp('    Z(f)')
  Multimeter : Subsystem  Tag=PoWeRsYsTeMmEaSuReMeNt  LoadFcn=powericonV2('psblcfmeas',gcb)  InitFcn=powericonV2('checksum',bdroot)  StopFcn=powericonV2('psbsignals')  mask(MultimeterPSB){PhasorSimulation=off, OutputType=Magnitude, sel=1, L=1, Gain=0, yselected={}, PSBOutputType=1, PSBequivalent=0, AxesSetting=[0,0.1,-100,100], Display=0, SavedBlockNames=-11}
      mask prompts: PhasorSimulation "Phasor simulation"; OutputType "Output signal"; sel "output selection"; L "vector length"; yselected "yout identifier"; PSBOutputType "Output type [1=PSB  0=simulink output]"; PSBequivalent "Equivalent circuit"; AxesSetting "Axes"; Display "Display Window"
      mask init:
      | NBS = length(sel);
      | switch OutputType
      | case 1
      |     OutputSelection  = [1:NBS];
      |     PhasorMode = [1:NBS];
      |     NormalMode = [NBS+1:2*NBS];
      | case 2
      |     for k=NBS+1:2*NBS;
      |         OutputSelection = [k,k+NBS];
      |     end
      |     PhasorMode = [1:2*NBS];
      |     NormalMode = [2*NBS+1:3*NBS];
      | case 3
      |     for k=2*NBS+1:3*NBS;
      |         OutputSelection = [k,k+NBS];
      |     end
      |     PhasorMode = [1:2*NBS];
      |     NormalMode = [2*NBS+1:3*NBS];
      | case 4
      |     OutputSelection  = [3*NBS+1:4*NBS];
      |     PhasorMode = [1:NBS];
      |     NormalMode = [NBS+1:2*NBS];
      | end
      | 
      | if PhasorSimulation
      |     SelectionMode = PhasorMode;
      | else
      |     SelectionMode = NormalMode;
      | end
      settings: CopyFcn=powericonV2('psblcfmeas',gcb,1)  DeleteFcn=if isempty(get_param(gcb,'UserData'));return;end; if get_param(gcb,'UserData')~=-1;close(get_param(gcb,'UserData'));end;  ModelCloseFcn=powericonV2('loadsavedata',gcs,'close')  OpenFcn=psbmultimeter(gcb)  CloseFcn=close(get_param(gcbh,'userdata'))
      mask StyleString: checkbox,popup(Complex|Real_Imag|Magnitude-angle|Magnitude),edit,edit,edit,edit,edit,edit,edit,edit,edit
      mask Display:
      | plot(0,0,100,100,[10,10,90,90,10],[90,10,10,90,90]);
      | disp(length(sel)*(sum(abs(Gain))>0))
  Three-Phase V-I Measurement : Subsystem  Tag=PoWeRsYsTeMmEaSuReMeNt  LoadFcn=powericonV2('psblfblk',gcbh,'3-Phase VI Measurement','');  InitFcn=powericonV2('checksum',bdroot)  mask(3-Phase VI Measurement){VChoice=phase-to-ground, ualv=off, labelV=V1, Vpu=off, Vbase=0, IChoice=yes, ualc=off, labelC=I1, Ppu=off, Pbase=0, OutputType=Complex, PhasorSimulation=off, PSBequivalent=0, PSBOutputType=11100}
      mask prompts: VChoice "Voltage measurement"; ualv "Use a label"; labelV "Signal label  (use a From block to collect signal)"; Vpu "Voltage  in pu"; Vbase "Base voltage (Vrms phase-phase) :"; IChoice "Current measurement"; ualc "Use a label"; labelC "Signal label  (use a From block to collect signal)"; Ppu "Currents in pu"; Pbase "Base power ( VA 3 phase)"; OutputType "Output signal :"; PhasorSimulation "Phasor simulation"; PSBequivalent "Equivalent circuit"
      mask help:
      | This block is used to measure three-phase voltages and currents in a circuit. When connected in series with a three-phase element, it return the three phase-to-ground voltages and line currents.
      |
      | The block can output the voltages and currents in per unit values or in volts and amperes. Check the appropriate boxes if you want to output the voltages and currents  in pu
      mask init:
      | powericonV2('psbcbtransfo',gcbh,'Three-phase measurements');
      | %	
      | if  Vpu
      |     xKv=1/(Vbase/sqrt(3)*sqrt(2));
      | else
      |     xKv=1;
      | end
      | if  Ppu
      |     xKi=1/(Pbase/Vbase/sqrt(3)*sqrt(2));
      | else
      |     xKi=1;
      | end
      | switch OutputType
      | case 1
      |     OutputSelection  = [1:6];
      |     PhasorModeV = [1:3];
      |     NormalModeV = [7:9];
      |     PhasorModeI = [4:6];
      |     NormalModeI = [10:12];
      |     Kv = xKv;
      |     Ki = xKi;
      | case 2
      |     OutputSelection = [7,13,8,14,9,15,10,16,11,17,12,18];
      |     PhasorModeV = [1:6];
      |     NormalModeV = [13:15];
      |     PhasorModeI = [7:12];
      |     NormalModeI = [16:18];
      |     Kv = xKv;
      |     Ki = xKi;
      | case 3
      |     OutputSelection = [13,19,14,20,15,21,16,22,17,23,18,24];
      |     PhasorModeV = [1:6];
      |     NormalModeV = [13:15];
      |     PhasorModeI = [7:12];
      |     NormalModeI = [16:18];
      |     Kv = [xKv 1 xKv 1 xKv 1];
      |     Ki = [xKi 1 xKi 1 xKi 1];
      | case 4
      |     OutputSelection  = [19:24];
      |     PhasorModeV = [1:3];
      |     NormalModeV = [7:9];
      |     PhasorModeI = [4:6];
      |     NormalModeI = [10:12];
      |     Kv = xKv;
      |     Ki = xKi;
      | end
      | if PhasorSimulation
      |     SelectionModeV = PhasorModeV;
      |     SelectionModeI = PhasorModeI;
      | else
      |     SelectionModeV = NormalModeV;
      |     SelectionModeI = NormalModeI;
      |     Kv = xKv;
      |     Ki = xKi;
      | end
      settings: CopyFcn=powericonV2('psblfblk',gcbh,'3-Phase VI Measurement','VerifyPhasor');  CloseFcn=%3phaseVImeasurement
      mask Help: web(psbhelp)
      mask StyleString: popup(no|phase-to-ground|phase-to-phase),checkbox,edit,checkbox,edit,popup(no|yes),checkbox,edit,checkbox,edit,popup(Complex|Real-Imag|Magnitude-Angle|Magnitude),checkbox,edit,edit
      mask CallbackString: powericonV2('psbcbtransfo',gcb,'Three-phase measurements');|powericonV2('psbcbtransfo',gcb,'Three-phase measurements');||powericonV2('psbcbtransfo',gcb,'Three-phase measurements');||powericonV2('psbcbtransfo',gcb,'Three-phase measurements');|powericonV2('psbcbtransfo',gcb,'Three-phase measurements');||powericonV2('psbcbtransfo',gcb,'Three-phase measurements');|||||
  Voltage Measurement : Subsystem  Tag=PoWeRsYsTeMmEaSuReMeNt  LoadFcn=powericonV2('psblcfmeas',gcb)  InitFcn=powericonV2('checksum',bdroot)  mask(Voltage Measurement){PhasorSimulation=off, OutputType=Magnitude, PSBOutputType=0, PSBequivalent=0}
      mask prompts: PhasorSimulation "Phasor simulation"; OutputType "Output signal :"; PSBOutputType "Output type [1=PSB  0=simulink output]"; PSBequivalent "Equivalent circuit"
      mask help: Ideal voltage measurement.
      mask init:
      | switch OutputType
      | case 1
      |     OutputSelection = 1;
      |     NormalMode = 2;
      |     PhasorMode = 1;
      | case 2
      |     OutputSelection =[2,3];
      |     NormalMode = 3;
      |     PhasorMode = [1,2];
      | case 3
      |     OutputSelection =[4,5];
      |     NormalMode = 3;
      |     PhasorMode = [1,2];
      | case 4
      |     OutputSelection =[4];
      |     NormalMode = 2;
      |     PhasorMode = 1;
      | end
      | %
      | if PhasorSimulation
      |     SelectionMode = PhasorMode;
      | else
      |     SelectionMode = NormalMode;
      | end
      settings: CopyFcn=powericonV2('psblcfmeas',gcb,1)  ModelCloseFcn=powericonV2('loadsavedata',gcs,'close')
      mask Help: web(psbhelp);
      mask StyleString: checkbox,popup(Complex|Real-Imag|Magnitude-Angle|Magnitude),edit,edit
